simulink model "quad_payload_model"  (R2019a)
settings: Solver=VariableStepAuto  StartTime=0.0  StopTime=20  MaxStep=0.05  RelTol=1e-3
values from neighbouring files (symbols this model uses):
  area = 0.1    [simulation_setup.m]
  b = 0.15    [simulation_setup.m]
  ba = 0.001    [simulation_setup.m]
  Cd = 1    [simulation_setup.m]
  fmax = 15    [simulation_setup.m]
  fmin = fmax*0.1    (= 1.5)    [simulation_setup.m]
  g = 9.81    [simulation_setup.m]
  J = (1/12)*M*(2*b)^2    (= 0.0075)    [simulation_setup.m]
  k1 = (2 * omega)*J    (= 0.4)    [simulation_setup.m]
  k2 = abs(( s * (s + a) ) / a)    [simulation_setup.m]
  k_x = acker(A_x,b_x,p_x)    [simulation_setup.m]
  k_z = acker(A_z,b_z,p_z)    [simulation_setup.m]
  L = 0.5    [simulation_setup.m]
  M = 1    [simulation_setup.m]
  m = 0.5    [simulation_setup.m]
  motor_t_const = 1/200    (= 0.005)    [simulation_setup.m]
  noise_freq_pos = 0.001    [simulation_setup.m]
  noise_freq_theta = 0.001    [simulation_setup.m]
  noise_freq_theta_dot = 0.001    [simulation_setup.m]
  noise_freq_vel = 0.001    [simulation_setup.m]
  rho = 1.225    [simulation_setup.m]
  theta_max = pi/4    (= 0.785398163397)    [simulation_setup.m]
libraries: simulink x9, dspfdesign x9, aerolibwind2 x1, aerolibutil x1
settings Model: Creator=johan  LastModifiedBy=johan

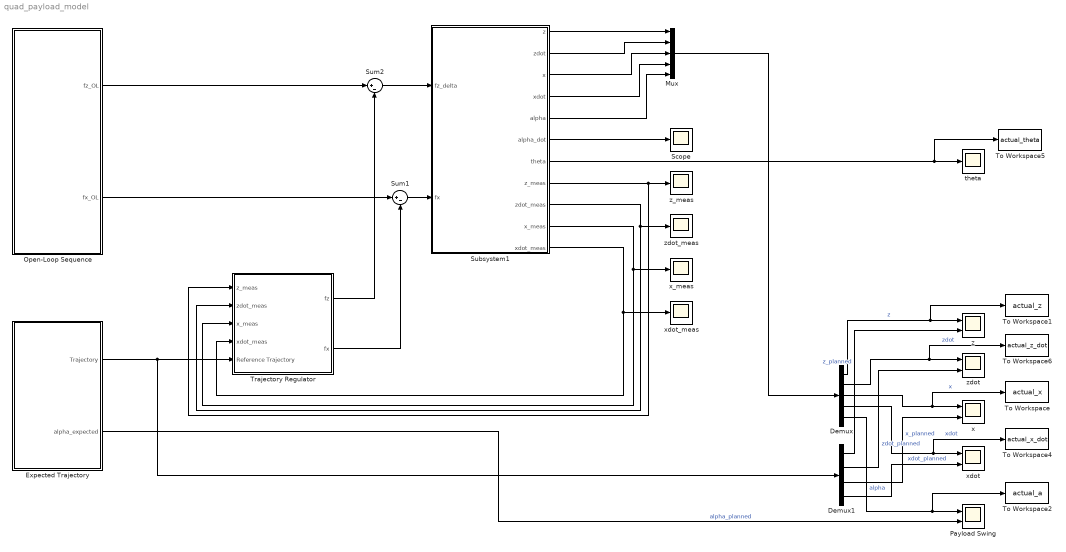
== system quad_payload_model ==
  Demux : Demux  Outputs=5
  Demux1 : Demux
  Expected Trajectory : Subsystem
  Mux : Mux  Inputs=5
  Open-Loop Sequence : Subsystem
  Payload Swing : Scope  NumInputPorts=2
  Scope : Scope
  Subsystem1 : Subsystem
  Sum1 : Sum  Inputs=|+-
  Sum2 : Sum  Inputs=|+-
  To Workspace : ToWorkspace  VariableName=actual_x  SaveFormat=Timeseries  SampleTime=-1
  To Workspace1 : ToWorkspace  VariableName=actual_z  SaveFormat=Timeseries  SampleTime=-1
  To Workspace2 : ToWorkspace  VariableName=actual_a  SaveFormat=Timeseries  SampleTime=-1
  To Workspace4 : ToWorkspace  VariableName=actual_x_dot  SaveFormat=Timeseries  SampleTime=-1
  To Workspace5 : ToWorkspace  VariableName=actual_theta  SaveFormat=Timeseries  SampleTime=-1
  To Workspace6 : ToWorkspace  VariableName=actual_z_dot  SaveFormat=Timeseries  SampleTime=-1
  Trajectory Regulator : Subsystem
  theta : Scope
  x : Scope  NumInputPorts=2
  x_meas : Scope
  xdot : Scope  NumInputPorts=2
  xdot_meas : Scope
  z : Scope  NumInputPorts=2
  z_meas : Scope
  zdot : Scope  NumInputPorts=2
  zdot_meas : Scope
  wires:
  Open-Loop Sequence/1(fz_OL) -> Sum2/1
  Open-Loop Sequence/2(fx_OL) -> Sum1/1
  Expected Trajectory/1(Trajectory) -> Demux1/1, Trajectory Regulator/5(Reference Trajectory)
  Trajectory Regulator/1(fz) -> Sum2/2
  Trajectory Regulator/2(fx) -> Sum1/2
  Sum2/1 -> Subsystem1/1(fz_delta)
  Sum1/1 -> Subsystem1/2(fx)
  Subsystem1/9(zdot_meas) -> Trajectory Regulator/2(zdot_meas), zdot_meas/1
  Subsystem1/8(z_meas) -> Trajectory Regulator/1(z_meas), z_meas/1
  Subsystem1/10(x_meas) -> Trajectory Regulator/3(x_meas), x_meas/1
  Subsystem1/11(xdot_meas) -> Trajectory Regulator/4(xdot_meas), xdot_meas/1
  Expected Trajectory/2(alpha_expected) -> Payload Swing/2  "alpha_planned"
  Subsystem1/1(z) -> Mux/1
  Subsystem1/2("zdot ") -> Mux/2
  Subsystem1/3(x) -> Mux/3
  Subsystem1/4(xdot) -> Mux/4
  Subsystem1/5(alpha) -> Mux/5
  Mux/1 -> Demux/1
  Demux/5 -> To Workspace2/1, Payload Swing/1  "alpha"
  Demux/1 -> To Workspace1/1, z/1  "z"
  Demux1/1 -> z/2  "z_planned"
  Demux/2 -> To Workspace6/1, zdot/1  "zdot"
  Demux1/2 -> zdot/2  "zdot_planned"
  Demux/3 -> To Workspace/1, x/1  "x"
  Demux1/3 -> x/2  "x_planned"
  Demux/4 -> To Workspace4/1, xdot/1  "xdot"
  Demux1/4 -> xdot/2  "xdot_planned"
  Subsystem1/7(theta) -> To Workspace5/1, theta/1
  Subsystem1/6(alpha_dot) -> Scope/1

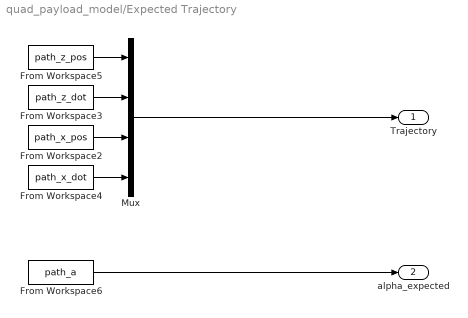
== system quad_payload_model/Expected Trajectory ==
  From Workspace2 : FromWorkspace  VariableName=path_x_pos  SampleTime=0
  From Workspace3 : FromWorkspace  VariableName=path_z_dot  SampleTime=0
  From Workspace4 : FromWorkspace  VariableName=path_x_dot  SampleTime=0
  From Workspace5 : FromWorkspace  VariableName=path_z_pos  SampleTime=0
  From Workspace6 : FromWorkspace  VariableName=path_a  SampleTime=0
  Mux : Mux
  Trajectory : Outport
  alpha_expected : Outport  Port=2
  wires:
  From Workspace5/1 -> Mux/1
  Mux/1 -> Trajectory/1
  From Workspace3/1 -> Mux/2
  From Workspace4/1 -> Mux/4
  From Workspace6/1 -> alpha_expected/1
  From Workspace2/1 -> Mux/3

== system quad_payload_model/Open-Loop Sequence ==
  From Workspace : FromWorkspace  VariableName=fz  SampleTime=0
  From Workspace1 : FromWorkspace  VariableName=fx  SampleTime=0
  fz_OL : Outport
  fx_OL : Outport  Port=2
  wires:
  From Workspace/1 -> fz_OL/1
  From Workspace1/1 -> fx_OL/1

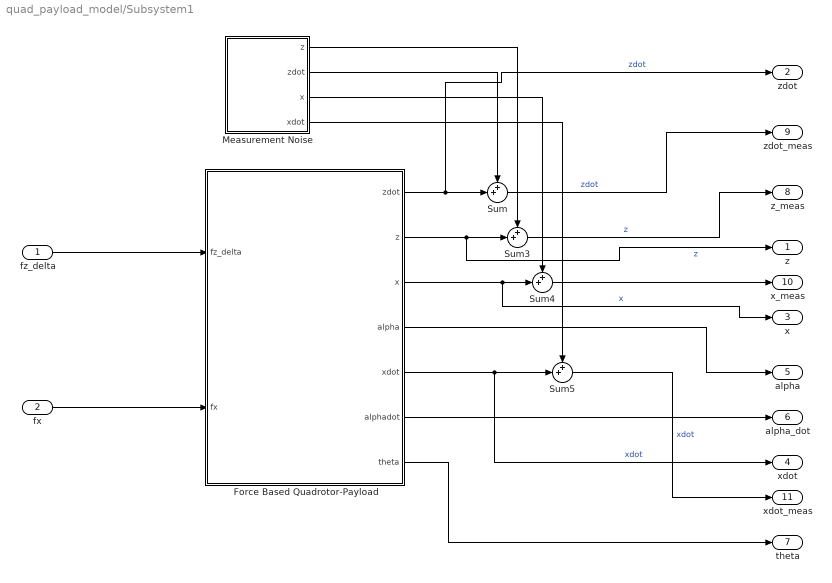
== system quad_payload_model/Subsystem1 ==
  fz_delta : Inport
  fx : Inport  Port=2
  Force Based Quadrotor-Payload : Subsystem
  Measurement Noise : Subsystem
  Sum{,3..5} (4 alike) : Sum  Inputs=++|
  z : Outport
  "zdot " : Outport  Port=2
  x : Outport  Port=3
  xdot : Outport  Port=4
  alpha : Outport  Port=5
  alpha_dot : Outport  Port=6
  theta : Outport  Port=7
  z_meas : Outport  Port=8
  zdot_meas : Outport  Port=9
  x_meas : Outport  Port=10
  xdot_meas : Outport  Port=11
  wires:
  Measurement Noise/2(zdot) -> Sum/1
  Measurement Noise/4(xdot) -> Sum5/1
  Measurement Noise/1(z) -> Sum3/1
  Force Based Quadrotor-Payload/3(x) -> x/1, Sum4/2  "x"
  Force Based Quadrotor-Payload/5(xdot) -> xdot/1, Sum5/2  "xdot"
  Force Based Quadrotor-Payload/2(z) -> z/1, Sum3/2  "z"
  Force Based Quadrotor-Payload/1(zdot) -> "zdot "/1, Sum/2  "zdot"
  Sum/1 -> zdot_meas/1  "zdot"
  Force Based Quadrotor-Payload/6(alphadot) -> alpha_dot/1
  Sum5/1 -> xdot_meas/1  "xdot"
  Force Based Quadrotor-Payload/4(alpha) -> alpha/1
  fz_delta/1 -> Force Based Quadrotor-Payload/1(fz_delta)
  Force Based Quadrotor-Payload/7(theta) -> theta/1
  Sum3/1 -> z_meas/1  "z"
  Measurement Noise/3(x) -> Sum4/1
  fx/1 -> Force Based Quadrotor-Payload/2(fx)
  Sum4/1 -> x_meas/1

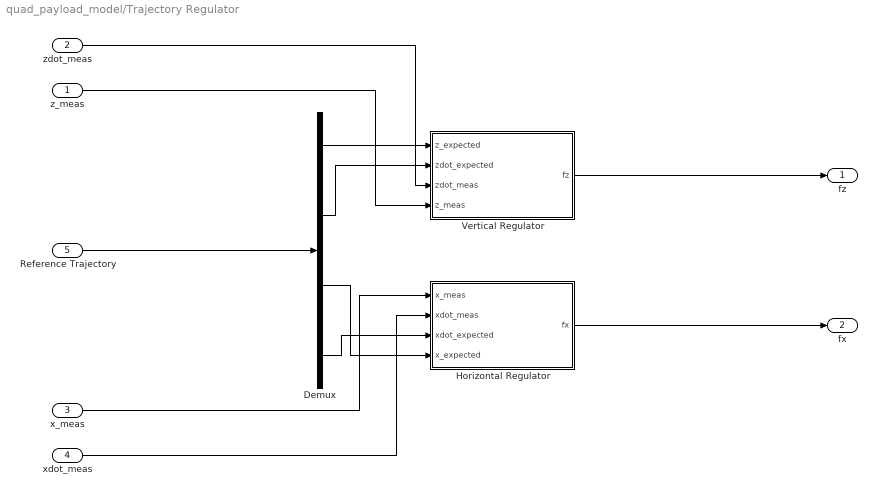
== system quad_payload_model/Trajectory Regulator ==
  z_meas : Inport
  zdot_meas : Inport  Port=2
  x_meas : Inport  Port=3
  xdot_meas : Inport  Port=4
  Reference Trajectory : Inport  Port=5
  Demux : Demux
  Horizontal Regulator : Subsystem
  Vertical Regulator : Subsystem
  fz : Outport
  fx : Outport  Port=2
  wires:
  zdot_meas/1 -> Vertical Regulator/3(zdot_meas)
  x_meas/1 -> Horizontal Regulator/1(x_meas)
  Vertical Regulator/1(fz) -> fz/1
  Reference Trajectory/1 -> Demux/1
  Horizontal Regulator/1(fx) -> fx/1
  Demux/2 -> Vertical Regulator/2(zdot_expected)
  xdot_meas/1 -> Horizontal Regulator/2(xdot_meas)
  z_meas/1 -> Vertical Regulator/4(z_meas)
  Demux/1 -> Vertical Regulator/1(z_expected)
  Demux/4 -> Horizontal Regulator/3(xdot_expected)
  Demux/3 -> Horizontal Regulator/4(x_expected)

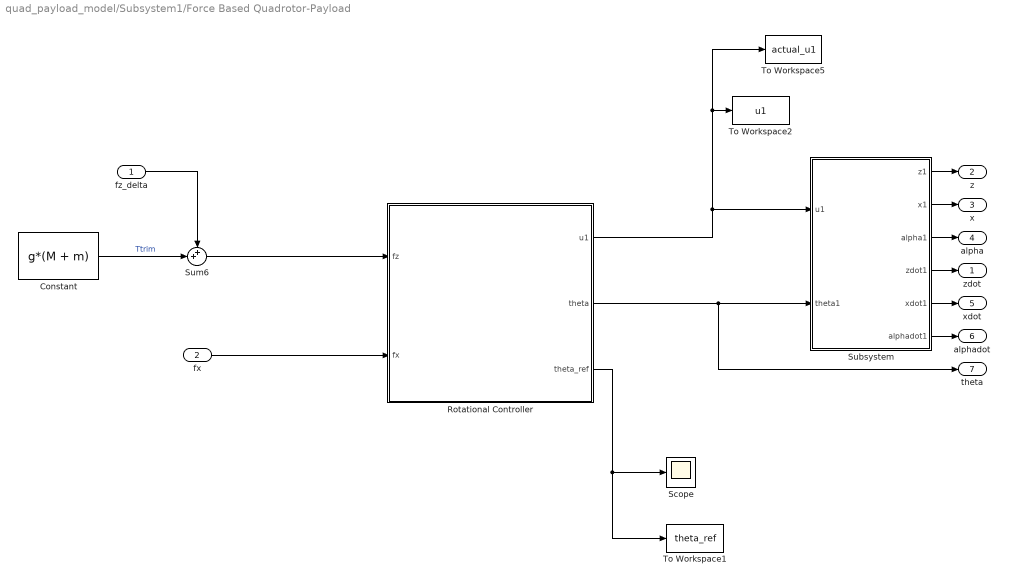
== system quad_payload_model/Subsystem1/Force Based Quadrotor-Payload ==
  fz_delta : Inport
  fx : Inport  Port=2
  Constant : Constant  Value=g*(M + m)
  Rotational Controller : Subsystem
  Scope : Scope
  Subsystem : Subsystem
  Sum6 : Sum  Inputs=++|
  To Workspace1 : ToWorkspace  VariableName=theta_ref  SampleTime=-1
  To Workspace2 : ToWorkspace  VariableName=u1  SampleTime=-1
  To Workspace5 : ToWorkspace  VariableName=actual_u1  SaveFormat=Timeseries  SampleTime=-1
  zdot : Outport
  z : Outport  Port=2
  x : Outport  Port=3
  alpha : Outport  Port=4
  xdot : Outport  Port=5
  alphadot : Outport  Port=6
  theta : Outport  Port=7
  wires:
  Rotational Controller/1(u1) -> To Workspace2/1, To Workspace5/1, Subsystem/1("u1 ")
  fx/1 -> Rotational Controller/2(fx)
  Subsystem/1(z1) -> z/1
  Rotational Controller/2(theta) -> Subsystem/2(theta1), theta/1
  Subsystem/5(xdot1) -> xdot/1
  Subsystem/3(alpha1) -> alpha/1
  Subsystem/2(x1) -> x/1
  Subsystem/6(alphadot1) -> alphadot/1
  Subsystem/4(zdot1) -> zdot/1
  Rotational Controller/3(theta_ref) -> Scope/1, To Workspace1/1
  Constant/1 -> Sum6/2  "Ttrim"
  Sum6/1 -> Rotational Controller/1(fz)
  fz_delta/1 -> Sum6/1

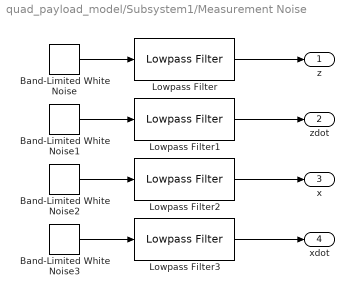
== system quad_payload_model/Subsystem1/Measurement Noise ==
  Band-Limited White Noise : simulink/Sources/Band-Limited White Noise  Cov=noise_p_pos  Ts=noise_freq_pos  seed=[3452345]
  Band-Limited White Noise1 : simulink/Sources/Band-Limited White Noise  Cov=noise_p_vel  Ts=noise_freq_vel  seed=[234]
  Band-Limited White Noise2 : simulink/Sources/Band-Limited White Noise  Cov=noise_p_pos  Ts=noise_freq_pos  seed=[34602]
  Band-Limited White Noise3 : simulink/Sources/Band-Limited White Noise  Cov=noise_p_vel  Ts=noise_freq_vel  seed=[256227]
  Lowpass Filter{,1..3} (4 alike) : dspfdesign/Lowpass Filter  FilterType=FIR  DesignForMinimumOrder=on  FilterOrder=50  PassbandFrequency=8e3  StopbandFrequency=12e3  PassbandRipple=0.1  StopbandAttenuation=80  InheritSampleRate=off  SampleRate=44100  SimulateUsing=Interpreted execution  roundingMode=Floor  coeffsDataTypeStr=fixdt(1,16)
  z : Outport
  zdot : Outport  Port=2
  x : Outport  Port=3
  xdot : Outport  Port=4
  wires:
  Band-Limited White Noise2/1 -> Lowpass Filter2/1
  Band-Limited White Noise1/1 -> Lowpass Filter1/1
  Lowpass Filter3/1 -> xdot/1
  Lowpass Filter2/1 -> x/1
  Lowpass Filter/1 -> z/1
  Band-Limited White Noise3/1 -> Lowpass Filter3/1
  Band-Limited White Noise/1 -> Lowpass Filter/1
  Lowpass Filter1/1 -> zdot/1

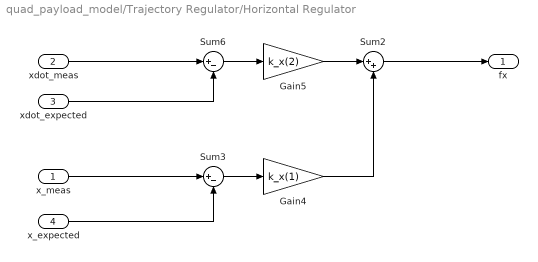
== system quad_payload_model/Trajectory Regulator/Horizontal Regulator ==
  x_meas : Inport
  xdot_meas : Inport  Port=2
  xdot_expected : Inport  Port=3
  x_expected : Inport  Port=4
  Gain4 : Gain  Gain=k_x(1)
  Gain5 : Gain  Gain=k_x(2)
  Sum2 : Sum  Inputs=|++
  Sum3 : Sum  Inputs=|+-
  Sum6 : Sum  Inputs=|+-
  fx : Outport
  wires:
  Sum3/1 -> Gain4/1
  Gain5/1 -> Sum2/1
  x_expected/1 -> Sum3/2
  Gain4/1 -> Sum2/2
  x_meas/1 -> Sum3/1
  xdot_expected/1 -> Sum6/2
  Sum2/1 -> fx/1
  Sum6/1 -> Gain5/1
  xdot_meas/1 -> Sum6/1

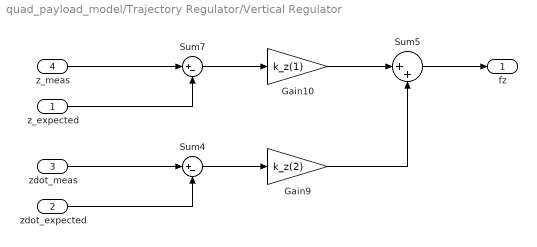
== system quad_payload_model/Trajectory Regulator/Vertical Regulator ==
  z_expected : Inport
  zdot_expected : Inport  Port=2
  zdot_meas : Inport  Port=3
  z_meas : Inport  Port=4
  Gain10 : Gain  Gain=k_z(1)
  Gain9 : Gain  Gain=k_z(2)
  Sum4 : Sum  Inputs=|+-
  Sum5 : Sum  Inputs=|++
  Sum7 : Sum  Inputs=|+-
  fz : Outport
  wires:
  Sum7/1 -> Gain10/1
  Gain9/1 -> Sum5/2
  Gain10/1 -> Sum5/1
  Sum4/1 -> Gain9/1
  Sum5/1 -> fz/1
  z_expected/1 -> Sum7/2
  zdot_meas/1 -> Sum4/1
  z_meas/1 -> Sum7/1
  zdot_expected/1 -> Sum4/2

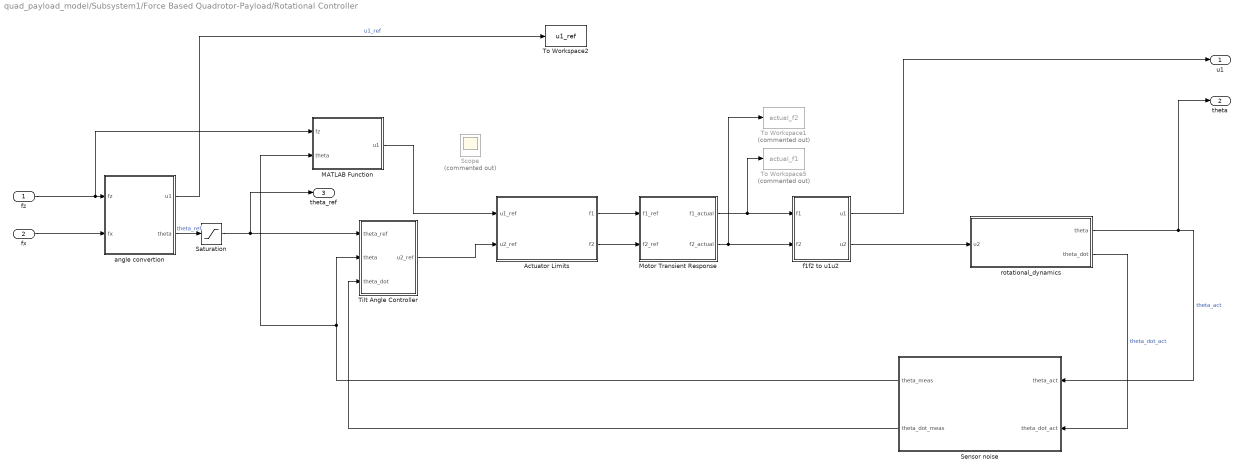
== system quad_payload_model/Subsystem1/Force Based Quadrotor-Payload/Rotational Controller ==
  fz : Inport
  fx : Inport  Port=2
  Actuator Limits : Subsystem
  MATLAB Function : MATLAB Function  TreatAsAtomicUnit=on
  Motor Transient Response : Subsystem
  Saturation : Saturate  UpperLimit=theta_max  LowerLimit=-theta_max
  Scope : Scope  Commented=on
  Sensor noise : Subsystem
  Tilt Angle Controller : Subsystem
  To Workspace1 : ToWorkspace  Commented=on  VariableName=actual_f2  SaveFormat=Timeseries  SampleTime=-1
  To Workspace2 : ToWorkspace  VariableName=u1_ref  SampleTime=-1
  To Workspace5 : ToWorkspace  Commented=on  VariableName=actual_f1  SaveFormat=Timeseries  SampleTime=-1
  angle convertion : MATLAB Function  TreatAsAtomicUnit=on
  f1f2 to u1u2 : Subsystem
  rotational_dynamics : Subsystem
  u1 : Outport
  theta : Outport  Port=2
  theta_ref : Outport  Port=3
  wires:
  fx/1 -> angle convertion/2(fx)
  angle convertion/2(theta) -> Saturation/1  "theta_ref"
  fz/1 -> MATLAB Function/1(fz), angle convertion/1(fz)
  angle convertion/1(u1) -> To Workspace2/1  "u1_ref"
  MATLAB Function/1(u1) -> Actuator Limits/1(u1_ref)
  Motor Transient Response/2(f2_actual) -> f1f2 to u1u2/2(f2), To Workspace1/1
  Motor Transient Response/1(f1_actual) -> f1f2 to u1u2/1(f1), To Workspace5/1
  Actuator Limits/1(f1) -> Motor Transient Response/1(f1_ref)
  Actuator Limits/2(f2) -> Motor Transient Response/2(f2_ref)
  rotational_dynamics/1(theta) -> theta/1, Sensor noise/1(theta_act)  "theta_act"
  f1f2 to u1u2/2(u2) -> rotational_dynamics/1(u2)
  Tilt Angle Controller/1(u2_ref) -> Actuator Limits/2(u2_ref)
  Sensor noise/1(theta_meas) -> Tilt Angle Controller/2(theta), MATLAB Function/2(theta)
  rotational_dynamics/2(theta_dot) -> Sensor noise/2(theta_dot_act)  "theta_dot_act"
  Sensor noise/2(theta_dot_meas) -> Tilt Angle Controller/3(theta_dot)
  Saturation/1 -> Tilt Angle Controller/1(theta_ref), theta_ref/1
  f1f2 to u1u2/1(u1) -> u1/1

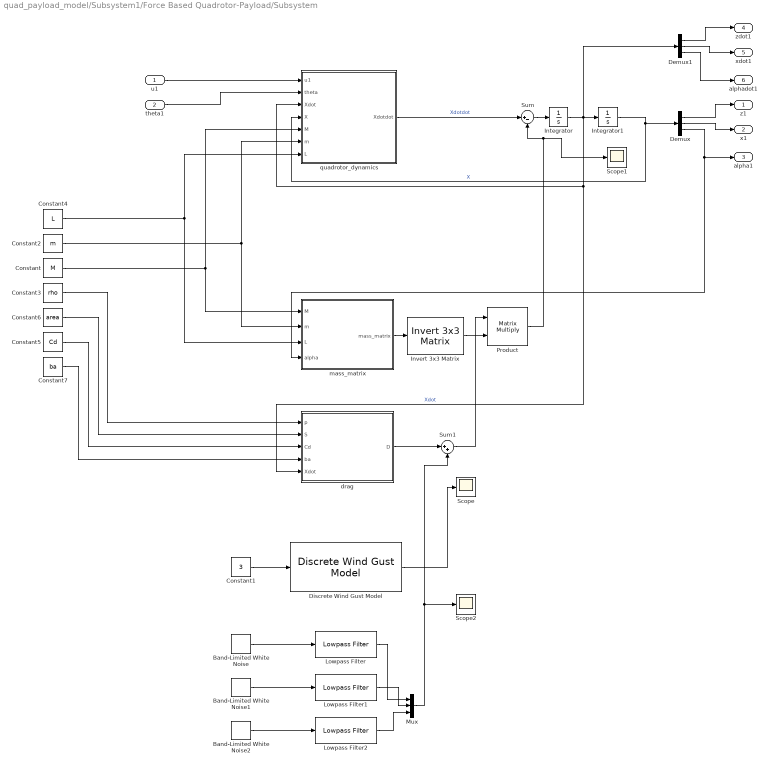
== system quad_payload_model/Subsystem1/Force Based Quadrotor-Payload/Subsystem ==
  "u1 " : Inport
  theta1 : Inport  Port=2
  Band-Limited White Noise : simulink/Sources/Band-Limited White Noise  Cov=[0.1]  Ts=0.1  seed=[23341]
  Band-Limited White Noise1 : simulink/Sources/Band-Limited White Noise  Cov=[0.1]  Ts=0.1  seed=[34563]
  Band-Limited White Noise2 : simulink/Sources/Band-Limited White Noise  Cov=[0.001*0]  Ts=0.1  seed=[02863]
  Constant : Constant  Value=M
  Constant1 : Constant  Value=3
  Constant2 : Constant  Value=m
  Constant3 : Constant  Value=rho
  Constant4 : Constant  Value=L
  Constant5 : Constant  Value=Cd
  Constant6 : Constant  Value=area
  Constant7 : Constant  Value=ba
  Demux : Demux  Outputs=3
  Demux1 : Demux  Outputs=3
  Discrete Wind Gust Model : aerolibwind2/Discrete Wind Gust Model  units=Metric (MKS)  Gx=on  Gy=on  Gz=on  t_0=1  d_m=[120 120 80]  v_m=[3.5 3.5 3.0]
      settings: SourceProductName=Aerospace Blockset
  Integrator : Integrator  InitialCondition=[0 0 0]
  Integrator1 : Integrator  InitialCondition=[0 0 0]
  Invert 3x3 Matrix : aerolibutil/Invert  3x3 Matrix
  Lowpass Filter : dspfdesign/Lowpass Filter  FilterType=FIR  DesignForMinimumOrder=on  FilterOrder=50  PassbandFrequency=8e3  StopbandFrequency=12e3  PassbandRipple=0.1  StopbandAttenuation=80  InheritSampleRate=off  SampleRate=44100  SimulateUsing=Interpreted execution  roundingMode=Floor  coeffsDataTypeStr=fixdt(1,16)
  Lowpass Filter1 : dspfdesign/Lowpass Filter  FilterType=FIR  DesignForMinimumOrder=on  FilterOrder=50  PassbandFrequency=8e3  StopbandFrequency=12e3  PassbandRipple=0.1  StopbandAttenuation=80  InheritSampleRate=off  SampleRate=44100  SimulateUsing=Interpreted execution  roundingMode=Floor  coeffsDataTypeStr=fixdt(1,16)
  Lowpass Filter2 : dspfdesign/Lowpass Filter  FilterType=FIR  DesignForMinimumOrder=on  FilterOrder=50  PassbandFrequency=8e3  StopbandFrequency=12e3  PassbandRipple=0.1  StopbandAttenuation=80  InheritSampleRate=off  SampleRate=44100  SimulateUsing=Interpreted execution  roundingMode=Floor  coeffsDataTypeStr=fixdt(1,16)
  Mux : Mux  Inputs=3
  Product : Product  Multiplication=Matrix(*)
  Scope : Scope
  Scope1 : Scope
  Scope2 : Scope
  Sum : Sum  Inputs=|+-
  Sum1 : Sum  Inputs=|++
  drag : MATLAB Function  TreatAsAtomicUnit=on
  mass_matrix : MATLAB Function  TreatAsAtomicUnit=on
  quadrotor_dynamics : MATLAB Function  TreatAsAtomicUnit=on
  z1 : Outport
  x1 : Outport  Port=2
  alpha1 : Outport  Port=3
  zdot1 : Outport  Port=4
  xdot1 : Outport  Port=5
  alphadot1 : Outport  Port=6
  wires:
  Demux/1 -> z1/1
  Constant/1 -> mass_matrix/1(M), quadrotor_dynamics/5(M)
  Demux1/1 -> zdot1/1
  theta1/1 -> quadrotor_dynamics/2(theta)
  Integrator1/1 -> Demux/1, quadrotor_dynamics/4(X)  "X"
  Product/1 -> Sum/2, Scope1/1
  Demux/2 -> x1/1
  Integrator/1 -> drag/5(Xdot), quadrotor_dynamics/3(Xdot), Demux1/1, Integrator1/1  "Xdot"
  Demux/3 -> alpha1/1, mass_matrix/4(alpha)
  Demux1/2 -> xdot1/1
  quadrotor_dynamics/1(Xdotdot) -> Sum/1  "Xdotdot"
  Sum/1 -> Integrator/1
  Demux1/3 -> alphadot1/1
  mass_matrix/1(mass_matrix) -> Invert 3x3 Matrix/1
  Invert 3x3 Matrix/1 -> Product/2
  "u1 "/1 -> quadrotor_dynamics/1(u1)
  Sum1/1 -> Product/1
  Constant7/1 -> drag/4(ba)
  Constant5/1 -> drag/3(Cd)
  Constant6/1 -> drag/2(S)
  Constant3/1 -> drag/1(p)
  Constant4/1 -> quadrotor_dynamics/7(L), mass_matrix/3(L)
  Constant2/1 -> mass_matrix/2(m), quadrotor_dynamics/6(m)
  drag/1(D) -> Sum1/1
  Discrete Wind Gust Model/1 -> Scope/1
  Constant1/1 -> Discrete Wind Gust Model/1
  Band-Limited White Noise/1 -> Lowpass Filter/1
  Mux/1 -> Scope2/1, Sum1/2
  Band-Limited White Noise1/1 -> Lowpass Filter1/1
  Band-Limited White Noise2/1 -> Lowpass Filter2/1
  Lowpass Filter1/1 -> Mux/2
  Lowpass Filter/1 -> Mux/1
  Lowpass Filter2/1 -> Mux/3

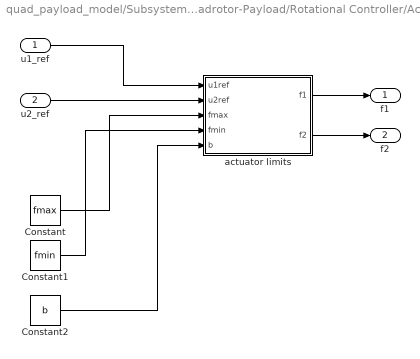
== system quad_payload_model/Subsystem1/Force Based Quadrotor-Payload/Rotational Controller/Actuator Limits ==
  u1_ref : Inport
  u2_ref : Inport  Port=2
  Constant : Constant  Value=fmax
  Constant1 : Constant  Value=fmin
  Constant2 : Constant  Value=b
  actuator limits : MATLAB Function  TreatAsAtomicUnit=on
  f1 : Outport
  f2 : Outport  Port=2
  wires:
  Constant2/1 -> actuator limits/5(b)
  u2_ref/1 -> actuator limits/2(u2ref)
  Constant/1 -> actuator limits/3(fmax)
  actuator limits/2(f2) -> f2/1
  Constant1/1 -> actuator limits/4(fmin)
  u1_ref/1 -> actuator limits/1(u1ref)
  actuator limits/1(f1) -> f1/1

== system quad_payload_model/Subsystem1/Force Based Quadrotor-Payload/Rotational Controller/Motor Transient Response ==
  f1_ref : Inport
  f2_ref : Inport  Port=2
  Transfer Fcn : TransferFcn  Numerator=[1/motor_t_const]  Denominator=[1 1/motor_t_const]
  Transfer Fcn2 : TransferFcn  Numerator=[1/motor_t_const]  Denominator=[1 1/motor_t_const]
  f1_actual : Outport
  f2_actual : Outport  Port=2
  wires:
  Transfer Fcn2/1 -> f2_actual/1
  f1_ref/1 -> Transfer Fcn/1
  Transfer Fcn/1 -> f1_actual/1
  f2_ref/1 -> Transfer Fcn2/1

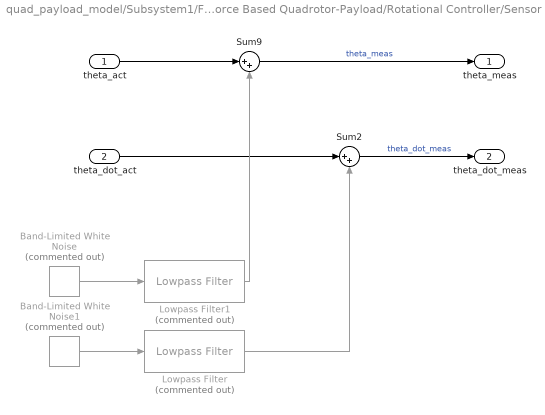
== system quad_payload_model/Subsystem1/Force Based Quadrotor-Payload/Rotational Controller/Sensor noise ==
  theta_act : Inport
  theta_dot_act : Inport  Port=2
  Band-Limited White Noise : simulink/Sources/Band-Limited White Noise  Commented=on  Cov=noise_p_theta  Ts=noise_freq_theta  seed=[14542]
  Band-Limited White Noise1 : simulink/Sources/Band-Limited White Noise  Commented=on  Cov=noise_p_theta_dot  Ts=noise_freq_theta_dot  seed=[56418]
  Lowpass Filter : dspfdesign/Lowpass Filter  Commented=on  FilterType=FIR  DesignForMinimumOrder=on  FilterOrder=50  PassbandFrequency=8e3  StopbandFrequency=12e3  PassbandRipple=0.1  StopbandAttenuation=80  InheritSampleRate=off  SampleRate=44100  SimulateUsing=Interpreted execution  roundingMode=Floor  coeffsDataTypeStr=fixdt(1,16)
  Lowpass Filter1 : dspfdesign/Lowpass Filter  Commented=on  FilterType=FIR  DesignForMinimumOrder=on  FilterOrder=50  PassbandFrequency=8e3  StopbandFrequency=12e3  PassbandRipple=0.1  StopbandAttenuation=80  InheritSampleRate=off  SampleRate=44100  SimulateUsing=Interpreted execution  roundingMode=Floor  coeffsDataTypeStr=fixdt(1,16)
  Sum2 : Sum  Inputs=|++
  Sum9 : Sum  Inputs=|++
  theta_meas : Outport
  theta_dot_meas : Outport  Port=2
  wires:
  theta_act/1 -> Sum9/1
  Sum2/1 -> theta_dot_meas/1  "theta_dot_meas"
  theta_dot_act/1 -> Sum2/1
  Sum9/1 -> theta_meas/1  "theta_meas"
  Band-Limited White Noise1/1 -> Lowpass Filter/1
  Band-Limited White Noise/1 -> Lowpass Filter1/1
  Lowpass Filter/1 -> Sum2/2
  Lowpass Filter1/1 -> Sum9/2

== system quad_payload_model/Subsystem1/Force Based Quadrotor-Payload/Rotational Controller/Tilt Angle Controller ==
  theta_ref : Inport
  theta : Inport  Port=2
  theta_dot : Inport  Port=3
  Gain1 : Gain  Gain=k1
  Gain2 : Gain  Gain=k2
  Sum : Sum  Inputs=|+-
  Sum1 : Sum  Inputs=|+-
  u2_ref : Outport
  wires:
  Sum/1 -> Gain2/1
  theta_dot/1 -> Sum1/2
  Sum1/1 -> Gain1/1
  theta_ref/1 -> Sum/1
  theta/1 -> Sum/2
  Gain2/1 -> Sum1/1
  Gain1/1 -> u2_ref/1  "u2_ref"

== system quad_payload_model/Subsystem1/Force Based Quadrotor-Payload/Rotational Controller/f1f2 to u1u2 ==
  f1 : Inport
  f2 : Inport  Port=2
  Constant : Constant  Value=b
  MATLAB Function1 : MATLAB Function  TreatAsAtomicUnit=on
  u1 : Outport
  u2 : Outport  Port=2
  wires:
  f2/1 -> MATLAB Function1/2(f2)
  f1/1 -> MATLAB Function1/1(f1)
  Constant/1 -> MATLAB Function1/3(b)
  MATLAB Function1/2(u2) -> u2/1  "u_2"
  MATLAB Function1/1(u1) -> u1/1

== system quad_payload_model/Subsystem1/Force Based Quadrotor-Payload/Rotational Controller/rotational_dynamics ==
  u2 : Inport
  Gain : Gain  Gain=1/J
  Integrator : Integrator
  Integrator1 : Integrator
  theta : Outport
  theta_dot : Outport  Port=2
  wires:
  Gain/1 -> Integrator1/1  "theta_ddot"
  Integrator1/1 -> theta_dot/1, Integrator/1  "theta_dot"
  Integrator/1 -> theta/1  "theta"
  u2/1 -> Gain/1

== matlab function quad_payload_model/Subsystem1/Force Based Quadrotor-Payload/Rotational Controller/angle convertion ==
  data: fz input; u1 output; fx input; theta output
function [u1,theta] = fcn(fz,fx)
u1 = sqrt(fz^2 + fx^2);
theta = atan(fx/fz);

== matlab function quad_payload_model/Subsystem1/Force Based Quadrotor-Payload/Rotational Controller/Actuator Limits/actuator limits ==
  data: u1ref input; u2ref input; f1 output; f2 output; fmax input; fmin input; b input
function [f1,f2]= act_limits(u1ref,u2ref, fmax, fmin, b)


if (u1ref > 2*fmax)
    u1ref = 2*fmax;
end
if (u1ref < 2*fmin)
    u1ref = 2*fmin;
end


fcommon = u1ref/2;
fdiff1 = fmax - fcommon;
fdiff2 = fcommon - fmin;

%Get max deviation from fcommon
if fdiff1 < fdiff2
    flim = fdiff1;
else
    flim = fdiff2;
end    
    
fdif = (u2ref)/(2*b);
if fdif > flim
    fdif = flim;
end

f1 = fcommon +fdif;

f2 = fcommon -fdif;
    

if (f1 > fmax)
    f1 = fmax;
end
if (f2 > fmax)
    f2 = fmax;
end
if (f1 < fmin)
    f1 = fmin;
end
if (f2 < fmin)
    f2 = fmin;
end

== matlab function quad_payload_model/Subsystem1/Force Based Quadrotor-Payload/Rotational Controller/f1f2 to u1u2/MATLAB Function1 ==
  data: f1 input; u1 output; f2 input; u2 output; b input
function [u1, u2]= system_inputs(f1,f2, b)

u1 = f1+ f2;
u2 = (f1-f2)*b;

== matlab function quad_payload_model/Subsystem1/Force Based Quadrotor-Payload/Rotational Controller/MATLAB Function ==
  data: fz input; u1 output; theta input
function u1 = fcn(fz,theta)

u1 = fz / cos(theta);

== matlab function quad_payload_model/Subsystem1/Force Based Quadrotor-Payload/Subsystem/drag ==
  data: p input; D output; S input; Cd input; ba input; Xdot input
function D = add_friction(p, S , Cd, ba, Xdot)
z_drag = (1/2)* p * Xdot(1) * Xdot(1) * S * Cd;
x_drag = (1/2)* p * Xdot(2) * Xdot(2) * S * Cd;
alpha_friction = ba * Xdot(3);

y = [z_drag x_drag alpha_friction];

D = y;

== matlab function quad_payload_model/Subsystem1/Force Based Quadrotor-Payload/Subsystem/mass_matrix ==
  data: M input; mass_matrix output; m input; L input; alpha input
function mass_matrix = calculate_M(M,m,L,alpha)

A = zeros([3,3]);
A(1,1) = M + m;
A(1,3) = m * L * sin (alpha);
A(2,2) = M + m;
A(2,3) = - m * L * cos(alpha);
A(3,1) = m * L * sin (alpha);
A(3,2) = -m * L * cos (alpha);
A(3,3) = m * L * L;

mass_matrix = A;

== matlab function quad_payload_model/Subsystem1/Force Based Quadrotor-Payload/Subsystem/quadrotor_dynamics ==
  data: u1 input; Xdotdot output; theta input; Xdot input; X input; M input; m input; L input

function Xdotdot = quadrotor_dynamics(u1, theta, Xdot, X, M, m, L)
g = 9.81;


alpha = X(3);
alphadot = Xdot(3);


fz = -g - ((m)/(M + m)) * L * cos(alpha )* alphadot^2;
fx = - (m/(M+m)) * L * sin(alpha )* alphadot^2;
gz = (1/(M + m)) * (cos(theta) + (m /(2 *M))* (cos(theta) - cos(theta - 2 * alpha)));
gx = (1/(M + m)) * (sin(theta) + (m /(2 *M))* (sin(theta) + sin(theta - 2 * alpha)));
ga = (1 / (M * L)) * sin(theta - alpha);

zdotdot = fz + gz*u1;
xdotdot = fx + gx*u1;
adotdot = ga*u1;

y = [zdotdot xdotdot adotdot];
Xdotdot = y;
